simulink model "ab"  (R2023b)
settings: configuration reference "VTOLConfiguration" (kept outside this file)
undefined symbols (not defined in the file): airspeed, CityMission, control, controlParams, ControlSampleTime, CriticalTiltAngle, ddx, ddy, ddz, DiscIntNeverNeededParam, dx, dy, dz, Earth, env, F, FixedWingMission, flightState, fractalcoef, FSState, FWControlParams, HoverMission, iniRoll, initPitch, iniYaw, Light, MIL, p, pitch, q, r, R_LOOKAHEAD, ReferenceFilterDen, ReferenceFilterNum, roll, SensorAAFiltDen, SensorAAFiltNum, tiltIni, TiltScheduleRate, TransitionMission, uavParam, UAVSampleTime, vIni, Vt, WGS84, windVel, X, xGround, Y, yaw, yGround, Z, zGround
libraries: slpidlib x37, simulink x10, uavalgslib x6, mbdriLib x4, robotcorelib x3, aerolibasang x2, aerolibwind2 x2, sharedtransform x2, simulink_extras x2, shared6dof x1, aerolibatmos2 x1, sensorgpslib x1
(part 1 of 7)
settings Model: DataDictionary=VTOLDynamicsData.sldd  Creator=The MathWorks, Inc.  LastModifiedBy=USER
settings ConfigSetRef: SourceName=VTOLConfiguration

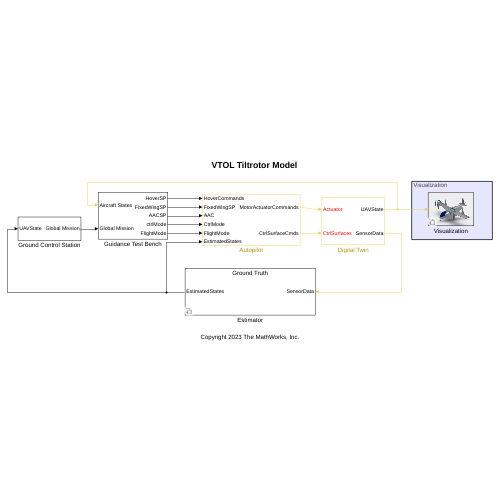
[thumbnail: Simulink's stored preview of the top-level diagram]
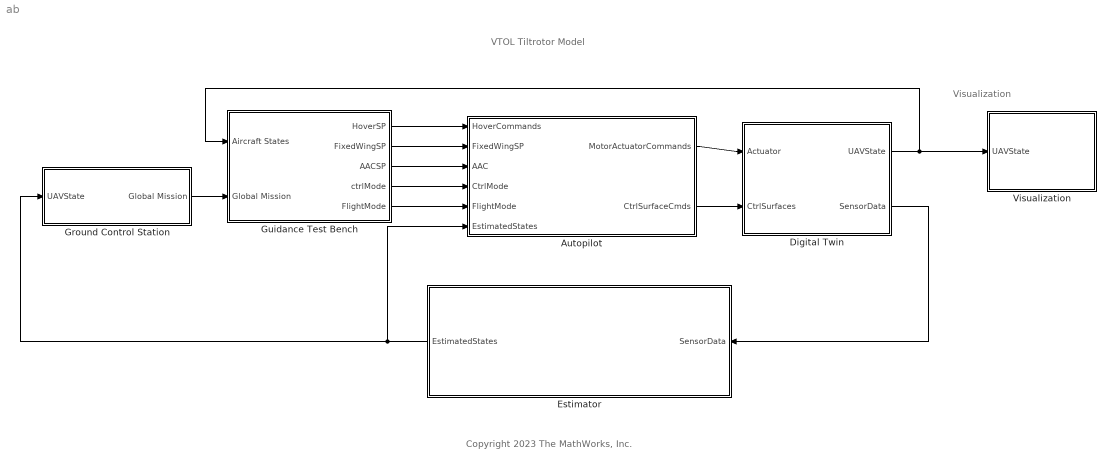
== system ab ==
  note: VTOL Tiltrotor Model
  note: Visualization
  note: Copyright 2023 The MathWorks, Inc.
  Autopilot : Subsystem
  Digital Twin : Subsystem
  Estimator : Subsystem  Variant=on
  Ground Control Station : Subsystem
  Guidance Test Bench : Subsystem
  Visualization : Subsystem  Variant=on  VariantControl=Visualization
      mask Display: image('TiltrotorVisualization.PNG'); % Use "Edit Image" on toolstrip to change.
  wires:
  Autopilot/1(MotorActuatorCommands) -> Digital Twin/1(Actuator)
  Autopilot/2(CtrlSurfaceCmds) -> Digital Twin/2(CtrlSurfaces)
  Digital Twin/2(SensorData) -> Estimator/1(SensorData)
  Guidance Test Bench/1(HoverSP) -> Autopilot/1(HoverCommands)
  Ground Control Station/1(Global Mission) -> Guidance Test Bench/2(Global Mission)
  Guidance Test Bench/2(FixedWingSP) -> Autopilot/2(FixedWingSP)
  Guidance Test Bench/3(AACSP) -> Autopilot/3(AAC)
  Guidance Test Bench/4(ctrlMode) -> Autopilot/4(CtrlMode)
  Guidance Test Bench/5(FlightMode) -> Autopilot/5(FlightMode)
  Digital Twin/1(UAVState) -> Guidance Test Bench/1(Aircraft States), Visualization/1(UAVState)
  Estimator/1(EstimatedStates) -> Autopilot/6(EstimatedStates), Ground Control Station/1(UAVState)

== system ab/Autopilot ==
  HoverCommands : Inport
  FixedWingSP : Inport  Port=2
  AAC : Inport  Port=3
  CtrlMode : Inport  Port=4
  FlightMode : Inport  Port=5
  EstimatedStates : Inport  Port=6
  Bus Selector : BusSelector  OutputSignals=inTransition
  Bus Selector1 : BusSelector  OutputSignals=TransitionCondition
  Bus Selector2 : BusSelector  OutputSignals=w1,w2,w3,w4
  Filter or Estimator : Subsystem
  Fixed Wing Controller : Subsystem  Variant=on  VariantControl=Fixed Wing Controller
  Manual Control : Subsystem
  Multicopter Controller : Subsystem
  Scheduler : Subsystem  SystemSampleTime=0.005
  Scope : Scope  NumInputPorts=4
  Scope1 : Scope
  Tilt Scheduler : Subsystem
  MotorActuatorCommands : Outport
  CtrlSurfaceCmds : Outport  Port=2
  wires:
  EstimatedStates/1 -> Filter or Estimator/1(SensorData)
  Multicopter Controller/1(MixerCommands) -> Scheduler/1(MotorCommands)
  Tilt Scheduler/1(TiltAngle) -> Scheduler/2(TiltSchedule)
  Fixed Wing Controller/1(Actuator) -> Scheduler/6(FixedWingActuators)
  CtrlMode/1 -> Bus Selector1/1, Fixed Wing Controller/2(Control Mode), Bus Selector/1
  Manual Control/1(AERT) -> Fixed Wing Controller/5(AERT)
  Scheduler/1(MotorActuatorCommands) -> Bus Selector2/1, MotorActuatorCommands/1
  Scheduler/2(CtrlSurfaceCommands) -> CtrlSurfaceCmds/1
  HoverCommands/1 -> Multicopter Controller/1(Hover Commands)
  FlightMode/1 -> Scope1/1, Tilt Scheduler/1(FlightMode)
  Filter or Estimator/1(States) -> Multicopter Controller/3(States), Fixed Wing Controller/1(States), Tilt Scheduler/2(States), Scheduler/4(States)
  AAC/1 -> Fixed Wing Controller/3(AAC SP)
  FixedWingSP/1 -> Fixed Wing Controller/4(FixedWingSP)
  [TransitionDone] -> Scheduler/5(TransitionDone)
  Tilt Scheduler/2(FlightState) -> Scheduler/3(FlightState)
  Bus Selector/1 -> Multicopter Controller/2(InTransition)  "<inTransition>"
  Bus Selector1/1 -> [TransitionDone]  "<TransitionCondition>"
  Bus Selector2/1 -> Scope/1  "<w1>"
  Bus Selector2/2 -> Scope/2  "<w2>"
  Bus Selector2/3 -> Scope/3  "<w3>"
  Bus Selector2/4 -> Scope/4  "<w4>"

== system ab/Digital Twin ==
  Actuator : Inport
  CtrlSurfaces : Inport  Port=2
  6DOF (Euler Angles)1 : shared6dof/6DOF (Euler Angles)  units=Metric (MKS)  mtype=Fixed  rep=Euler Angles  xme_0=[xGround, yGround, zGround]  Vm_0=[vIni 0 0]  eul_0=[iniRoll initPitch iniYaw]  pm_0=[0 0 0]  mass_0=6.031  mass_e=0.5  mass_f=2.0  inertia=[uavParam.geom.Ixx 0 0; 0 uavParam.geom.Iyy 0; 0 0 uavParam.geom.Izz]  inertia_e=eye(3)  inertia_f=2*eye(3)  k_quat=1.0  vre_flag=on  abi_flag=on  aMode=0  xme_statename=''  Vm_statename=''  eul_statename=''  quat_statename=''  pm_statename=''  mass_statename=''
  Bus Selector : BusSelector  OutputSignals=RotorParameters.w1,RotorParameters.w2,RotorParameters.w3,RotorParameters.w4
  Force and Moments : Subsystem
  Ground Truth Bus : Subsystem
  Scope : Scope  NumInputPorts=4
  Terminator : Terminator
  Variant Subsystem : Subsystem  Variant=on  VariantControl=Choice
  UAVState : Outport
  SensorData : Outport  Port=2
  wires:
  Force and Moments/1(F) -> 6DOF (Euler Angles)1/1
  Force and Moments/2(M) -> 6DOF (Euler Angles)1/2
  Actuator/1 -> Force and Moments/1(Actuator)
  CtrlSurfaces/1 -> Force and Moments/2(CtrlSurfaces)
  6DOF (Euler Angles)1/1 -> Ground Truth Bus/1(Ve)  "Ve"
  6DOF (Euler Angles)1/2 -> Ground Truth Bus/2(Xe)  "Xe"
  6DOF (Euler Angles)1/3 -> Ground Truth Bus/3(Euler)  "Euler"
  6DOF (Euler Angles)1/4 -> Ground Truth Bus/4(DCMbe)  "DCMbe"
  6DOF (Euler Angles)1/5 -> Ground Truth Bus/5(Vb)  "Vb"
  6DOF (Euler Angles)1/6 -> Ground Truth Bus/6(pqr)  "pqr"
  6DOF (Euler Angles)1/7 -> Terminator/1
  6DOF (Euler Angles)1/8 -> Ground Truth Bus/7(Abb)  "Abb"
  Force and Moments/3(RotorParams) -> Ground Truth Bus/9(RotorParams)  "RotorParams"
  Force and Moments/4(AirData) -> Ground Truth Bus/10(AirData)
  Variant Subsystem/1(SensorData) -> SensorData/1
  6DOF (Euler Angles)1/9 -> Ground Truth Bus/8(Abe)
  Ground Truth Bus/1(Ground Truth) -> Bus Selector/1, UAVState/1, Force and Moments/3(States), Variant Subsystem/1(UAVStates)  "Ground Truth"
  Bus Selector/1 -> Scope/1  "<w1>"
  Bus Selector/2 -> Scope/2  "<w2>"
  Bus Selector/3 -> Scope/3  "<w3>"
  Bus Selector/4 -> Scope/4  "<w4>"

== system ab/Estimator ==
  SensorData : Inport
  Estimation Filter : Subsystem  VariantControl=SensorType==1
  Ground Truth : Subsystem  VariantControl=SensorType==0
  EstimatedStates : Outport

== system ab/Ground Control Station ==
  UAVState : Inport
  Get Flight Mission : Subsystem  Variant=on  VariantControlMode=label  LabelModeActiveChoice=useQGC==0
  Global Mission : Outport
  wires:
  Get Flight Mission/1("Mission ") -> Global Mission/1
  UAVState/1 -> Get Flight Mission/1(UAVState)

== system ab/Guidance Test Bench ==
  Aircraft States : Inport
  Global Mission : Inport  Port=2
  ControlType : Subsystem  Variant=on  VariantControl=Choice
  Rate Transition : RateTransition  OutPortSampleTime=0.005
  "Reference Tracking " : Subsystem
      settings: PortSchema="{\"entries\":[{\"content\":{\"sides\":[{\"content\":{\"connectorIds\":[\"In1\"]},\"type\":\"ConnectorPlacement.EquallySpacedRectSide\",\"uuid\":\"259d5f1e-a362-4dc0-8429-ef92dd781b31\"},{\"content\":{\"connectorIds\":[\"In2\",\"In3\"],\"side\":\"RIGHT\"},\"type\":\"ConnectorPlacement.EquallySpacedRectSide\",\"uuid\":\"8f699bfb-ab92-4bfa-94de-3c6c350a8a94\"},{\"content\":{\"connectorIds\":[],\"side\":\"TOP\"},\"type\":\"ConnectorPlacement.EquallySpacedRectSide\",\"uuid\":\"95dbffc6-e5b7-446a-adcb-afa0cff8c552\"}]},\"type\":\"ConnectorPlacement.EquallySpacedConnector\",\"uuid\":\"e657b5d9-4fa5-41f8-85e3-18a1074ff1cd\"}],\"packageUris\":[\"http://schema.mathworks.com/mf0/Connector/R2020b\"],\"version\":\"1.0\"}"
  HoverSP : Outport
  FixedWingSP : Outport  Port=2
  AACSP : Outport  Port=3
  ctrlMode : Outport  Port=4
  FlightMode : Outport  Port=5
  wires:
  Aircraft States/1 -> Rate Transition/1
  ControlType/1(HoverCmds) -> "Reference Tracking "/2(Position Command), HoverSP/1
  Global Mission/1 -> ControlType/2(Global Mission)
  ControlType/2(FixedWingSP) -> FixedWingSP/1
  ControlType/5(FlightMode) -> FlightMode/1
  ControlType/4(ctrlMode) -> ctrlMode/1
  ControlType/3(AACSP) -> "Reference Tracking "/3(AAC Commands), AACSP/1
  Rate Transition/1 -> "Reference Tracking "/1(State), ControlType/1(Aircraft States)

== system ab/Visualization ==
  UAVState : Inport
  No Visualization : Subsystem  VariantControl=Visualization==0
  Photorealistic : Subsystem  VariantControl=Visualization==2
  Visualization : Subsystem  VariantControl=Visualization==1

== system ab/Autopilot/Filter or Estimator ==
  SensorData : Inport
  States : Outport
  wires:
  SensorData/1 -> States/1

== system ab/Autopilot/Fixed Wing Controller ==
  States : Inport
  Control Mode : Inport  Port=2
  AAC SP : Inport  Port=3
  FixedWingSP : Inport  Port=4
  AERT : Inport  Port=5
  Fixed Wing Controller Simulation : Subsystem  VariantControl=TuningMode == 0
  Fixed Wing Controller Tuning : Subsystem  VariantControl=TuningMode ~= 0
  Actuator : Outport

== system ab/Autopilot/Manual Control ==
  Bus Creator : BusCreator  Inputs=4
  Constant{,1..3} (4 alike) : Constant  Value=0
  AERT : Outport
  wires:
  Constant/1 -> Bus Creator/1  "aileron"
  Constant1/1 -> Bus Creator/2  "throttle"
  Constant2/1 -> Bus Creator/3  "elevator"
  Constant3/1 -> Bus Creator/4  "rudder"
  Bus Creator/1 -> AERT/1

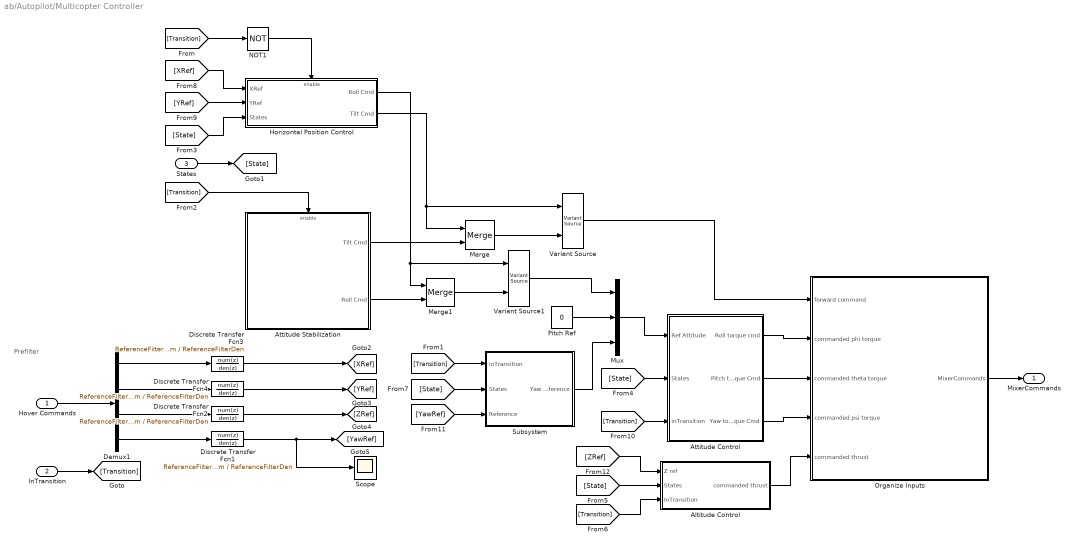
== system ab/Autopilot/Multicopter Controller ==
  note: Prefilter
  Hover Commands : Inport
  InTransition : Inport  Port=2
  States : Inport  Port=3
  Altitude Control : Subsystem
  Attitude Control : Subsystem  Variant=on  VariantControlMode=label  VariantControl=Choice  LabelModeActiveChoice=AttitudeControl==1
  Attitude Stabilization : Subsystem  TreatAsAtomicUnit=on
  Demux1 : Demux
  Discrete Transfer Fcn{1..4} (4 alike) : DiscreteTransferFcn  Numerator=ReferenceFilterNum  Denominator=ReferenceFilterDen
  Horizontal Position Control : Subsystem  TreatAsAtomicUnit=on
  Merge : Merge
  Merge1 : Merge
  Mux : Mux  Inputs=3
  NOT1 : Logic  Operator=NOT  IconShape=distinctive  AllPortsSameDT=off  OutDataTypeStr=boolean
  Organize Inputs : Subsystem
  Pitch Ref : Constant  Value=0
  Scope : Scope
  Subsystem : Subsystem
  Variant Source : VariantSource
  Variant Source1 : VariantSource
  MixerCommands : Outport
  wires:
  [Transition] -> NOT1/1
  [State] -> Horizontal Position Control/3(States)
  Variant Source1/1 -> Mux/1
  States/1 -> [State]
  Hover Commands/1 -> Demux1/1
  InTransition/1 -> [Transition]
  NOT1/1 -> Horizontal Position Control/Enable
  [YRef] -> Horizontal Position Control/2(YRef)
  [XRef] -> Horizontal Position Control/1(XRef)
  Attitude Control/1(Roll torque cmd) -> Organize Inputs/2(commanded phi torque)
  [Transition] -> Attitude Stabilization/Enable
  Demux1/3 -> Discrete Transfer Fcn2/1
  Demux1/1 -> Discrete Transfer Fcn3/1
  [State] -> Altitude Control/2(States)
  Demux1/2 -> Discrete Transfer Fcn4/1
  Discrete Transfer Fcn3/1 -> [XRef]
  Demux1/4 -> Discrete Transfer Fcn1/1
  Horizontal Position Control/1(Roll Cmd) -> Variant Source1/1, Merge1/1
  Horizontal Position Control/2(Tilt Cmd) -> Merge/1, Variant Source/1
  Attitude Control/3(Yaw torque Cmd) -> Organize Inputs/4(commanded psi torque)
  Attitude Stabilization/1(Tilt Cmd) -> Merge/2
  Attitude Control/2(Pitch torque Cmd) -> Organize Inputs/3(commanded theta torque)
  Attitude Stabilization/2(Roll Cmd) -> Merge1/2
  Discrete Transfer Fcn4/1 -> [YRef]
  Merge/1 -> Variant Source/2
  Merge1/1 -> Variant Source1/2
  [Transition] -> Subsystem/1(inTransition)
  [State] -> Subsystem/2(States)
  [YawRef] -> Subsystem/3(Reference)
  Variant Source/1 -> Organize Inputs/1(forward command)
  Pitch Ref/1 -> Mux/2
  Subsystem/1(Yaw Reference) -> Mux/3
  Mux/1 -> Attitude Control/1(Ref Attitude)
  [State] -> Attitude Control/2(States)
  [Transition] -> Attitude Control/3(inTransition)
  [ZRef] -> Altitude Control/1(Z ref)
  [Transition] -> Altitude Control/3(InTransition)
  Altitude Control/1(commanded thrust) -> Organize Inputs/5(commanded thrust)
  Organize Inputs/1(MixerCommands) -> MixerCommands/1
  Discrete Transfer Fcn1/1 -> Scope/1, [YawRef]
  Discrete Transfer Fcn2/1 -> [ZRef]

== system ab/Autopilot/Scheduler ==
  MotorCommands : Inport
  TiltSchedule : Inport  Port=2
  FlightState : Inport  Port=3  OutDataTypeStr=Enum: flightState
  States : Inport  Port=4
  TransitionDone : Inport  Port=5
  FixedWingActuators : Inport  Port=6
  Subsystem : Subsystem  ReferencedSubsystem=FixedWingScheduler
  Subsystem1 : Subsystem  ReferencedSubsystem=MulticopterScheduler
  MotorActuatorCommands : Outport
  CtrlSurfaceCommands : Outport  Port=2  VectorParamsAs1DForOutWhenUnconnected=off
  wires:
  Subsystem/1 -> Subsystem1/2, CtrlSurfaceCommands/1
  FlightState/1 -> Subsystem/1, Subsystem1/1  "Flight State"
  TiltSchedule/1 -> Subsystem1/4
  Subsystem1/1 -> MotorActuatorCommands/1
  MotorCommands/1 -> Subsystem1/3
  FixedWingActuators/1 -> Subsystem/2
  TransitionDone/1 -> Subsystem/3, Subsystem1/5  "Transition Done"
  States/1 -> Subsystem1/6

== system ab/Autopilot/Tilt Scheduler ==
  note: Forward Transition Tilt Mode Manager
  note: Back Transition Tilt Mode Manager
  FlightMode : Inport
  States : Inport  Port=2
  Back Transition Scheduler : Subsystem
  Forward Transition Scheduler : Subsystem
  TiltAngle : Outport
  FlightState : Outport  Port=2
  wires:
  States/1 -> Back Transition Scheduler/3(States)
  Back Transition Scheduler/1(TiltAngle) -> TiltAngle/1
  FlightMode/1 -> Back Transition Scheduler/2(FlightMode), Forward Transition Scheduler/1(FlightMode)
  Forward Transition Scheduler/1(FlightState) -> FlightState/1
  Forward Transition Scheduler/2(Tilt Schedule) -> Back Transition Scheduler/1(Tilt Schedule)

== system ab/Digital Twin/Force and Moments ==
  Actuator : Inport
  CtrlSurfaces : Inport  Port=2
  States : Inport  Port=3
  Add : Sum  Inputs=++++
  Add1 : Sum
  AeroSwitch : Constant
  Aerodynamic Drag : Subsystem
  Aerodynamic Forces : Subsystem
  Bus Selector : BusSelector  OutputSignals=DCMbe,Vb
  Bus Selector3 : BusSelector  OutputSignals=Xe,Euler
  Constant4 : Constant  Value=0
  Constant5 : Constant  Value=0
  Gravity : Subsystem
  Propulsion : Subsystem
  Switch : Switch  Criteria=u2 > Threshold  SaturateOnIntegerOverflow=off  InputSameDT=off
  Switch1 : Switch  Criteria=u2 > Threshold  SaturateOnIntegerOverflow=off  InputSameDT=off
  Weather Model : Subsystem  Variant=on  VariantControl=Weather Model
  F : Outport
  M : Outport  Port=2
  RotorParams : Outport  Port=3
  AirData : Outport  Port=4
  wires:
  Bus Selector/1 -> Gravity/1(DCM_be), Aerodynamic Drag/1(DCM_be)  "<DCMbe>"
  Propulsion/3(F) -> Add/1
  Gravity/1(F_g) -> Add/2  "Gravity Force"
  Aerodynamic Drag/1(F_d) -> Add/4  "Drag Force"
  Bus Selector/2 -> Aerodynamic Drag/2(Vb)  "<Vb>"
  Add/1 -> F/1
  States/1 -> Bus Selector3/1, Bus Selector/1, Aerodynamic Forces/4(UAVState), Propulsion/2(States)  "States"
  CtrlSurfaces/1 -> Aerodynamic Forces/3(CtrlSurfaces)
  Add1/1 -> M/1
  Propulsion/2(M) -> Add1/2
  [AeroForce] -> Add/3  "Aerodynamic Force"
  Aerodynamic Forces/2(F) -> Switch/1
  Switch/1 -> [AeroForce]
  Constant4/1 -> Switch/3
  AeroSwitch/1 -> Switch/2, Switch1/2
  Constant5/1 -> Switch1/3
  Switch1/1 -> Add1/1, [AeroMoment]
  Aerodynamic Forces/3(M) -> Switch1/1
  Actuator/1 -> Propulsion/1(Actuator)
  Propulsion/1(RotorParameters) -> RotorParams/1
  Aerodynamic Forces/1(AirData) -> AirData/1, Weather Model/1(AirData)  "Air Data"
  Bus Selector3/1 -> Weather Model/2(Xe)  "<Xe>"
  Bus Selector3/2 -> Weather Model/3(Euler)  "<Euler>"
  Weather Model/1(Wind_e) -> Aerodynamic Forces/1(Wind_e)
  Weather Model/2(Rho) -> Aerodynamic Forces/2(Rho)

== system ab/Digital Twin/Ground Truth Bus ==
  Ve : Inport
  Xe : Inport  Port=2
  Euler : Inport  Port=3
  DCMbe : Inport  Port=4
  Vb : Inport  Port=5
  pqr : Inport  Port=6
  Abb : Inport  Port=7
  Abe : Inport  Port=8
  RotorParams : Inport  Port=9
  AirData : Inport  Port=10
  Bus Creator : BusCreator  Inputs=13
  Bus Selector : BusSelector  OutputSignals=airspeed
  Direction Cosine Matrix to Quaternions : sharedtransform/Direction Cosine Matrix  to Quaternions  aMode=0  action=None  tolerance=eps(2)
      settings: LibrarySourceBlock=|
      | aerolibtransform2/Direction Cosine Matrix
      | to Quaternions
  MATLAB Function1 : MATLAB Function  TreatAsAtomicUnit=on
  Ground Truth : Outport
  wires:
  pqr/1 -> Bus Creator/6
  Xe/1 -> Bus Creator/2
  Bus Creator/1 -> Ground Truth/1
  DCMbe/1 -> Direction Cosine Matrix to Quaternions/1, Bus Creator/4
  Euler/1 -> Bus Creator/3
  Vb/1 -> Bus Creator/5
  Abb/1 -> Bus Creator/7
  AirData/1 -> Bus Selector/1
  Bus Selector/1 -> Bus Creator/9  "<airspeed>"
  Direction Cosine Matrix to Quaternions/1 -> Bus Creator/10  "q"
  RotorParams/1 -> Bus Creator/8  "RotorParameters"
  Abe/1 -> Bus Creator/11  "Abe"
  MATLAB Function1/2(gndSpeed) -> Bus Creator/13  "gndspeed"
  MATLAB Function1/1(course) -> Bus Creator/12  "course"
  Ve/1 -> MATLAB Function1/1(vxyz), Bus Creator/1

== system ab/Digital Twin/Variant Subsystem ==
  UAVStates : Inport
  No Sensors : Subsystem  VariantControl=SensorType==0
  Sensors : Subsystem  VariantControl=SensorType==1
  SensorData : Outport

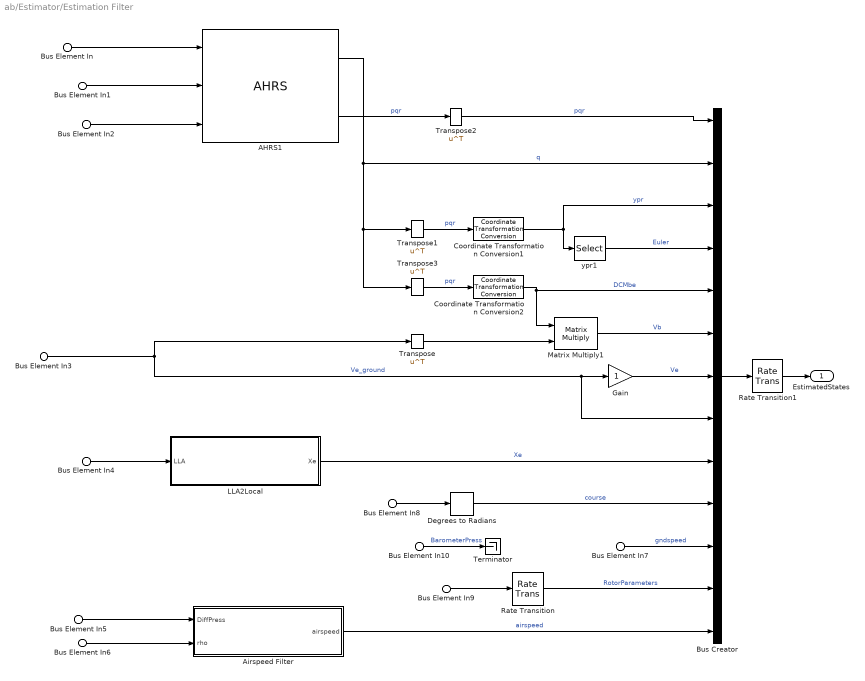
== system ab/Estimator/Estimation Filter ==
  Bus Element In : Inport  PortName=SensorData  Element=Abb
  Bus Element In1 : Inport  PortName=SensorData  Element=Gyro
  Bus Element In2 : Inport  PortName=SensorData  Element=Mag
  Bus Element In3 : Inport  PortName=SensorData  Element=GPSVelocity
  Bus Element In4 : Inport  PortName=SensorData  Element=LLA
  Bus Element In6 : Inport  PortName=SensorData  Element=rho
  Bus Element In5 : Inport  PortName=SensorData  Element=DiffPress
  Bus Element In7 : Inport  PortName=SensorData  Element=GPSGroundSpeed
  Bus Element In8 : Inport  PortName=SensorData  Element=GPSCourse
  Bus Element In9 : Inport  PortName=SensorData  Element=RotorParameters
  Bus Element In10 : Inport  PortName=SensorData  Element=BarometerPress
  AHRS1 : mspfiltlib/AHRS  DispRefFrame=NED  DecimationFactor=1  InitialProcessNoise=ahrsfilter.defaultProcessNoise  OrientationFormat=quaternion  SimulateUsing=Code generation  AccelerometerNoise=0.0001924722  GyroscopeNoise=9.1385e-5  MagnetometerNoise=0.1  GyroscopeDriftNoise=3.0462e-13  LinearAccelerationNoise=0.0096236100000000012  MagneticDisturbanceNoise=0.5  LinearAccelerationDecayFactor=0.998  MagneticDisturbanceDecayFactor=0.5  ExpectedMagneticFieldStrength=40
  Airspeed Filter : Subsystem
  Bus Creator : BusCreator  Inputs=13
  Coordinate Transformation Conversion1 : robotcorelib/Coordinate Transformation Conversion  InputRepresentation=Quaternion  InputEulerSequence=ZYX  ShowTrVecInputPort=on  OutputRepresentation=Euler Angles  OutputEulerSequence=ZYX  ShowTrVecOutputPort=on  SimulateUsing=Interpreted execution
      settings: LibrarySourceBlock=navlib/Utilities/Coordinate Transformation Conversion
  Coordinate Transformation Conversion2 : robotcorelib/Coordinate Transformation Conversion  InputRepresentation=Quaternion  InputEulerSequence=ZYX  ShowTrVecInputPort=on  OutputRepresentation=Rotation Matrix  OutputEulerSequence=ZYX  ShowTrVecOutputPort=on  SimulateUsing=Interpreted execution
      settings: LibrarySourceBlock=navlib/Utilities/Coordinate Transformation Conversion
  Degrees to Radians : simulink_extras/Transformations/Degrees to Radians
  Gain : Gain
  LLA2Local : Subsystem
  Matrix Multiply1 : Product  Multiplication=Matrix(*)
  Rate Transition : RateTransition  OutPortSampleTime=0.001
  Rate Transition1 : RateTransition
  Terminator : Terminator
  Transpose{,1..3} (4 alike) : Math  Operator=transpose
  ypr1 : Selector  InputPortWidth=3  IndexOptions=Index vector (dialog)  Indices=[3 2 1]  OutputSizes=1
  EstimatedStates : Outport
  wires:
  AHRS1/2 -> Transpose2/1  "pqr"
  Bus Element In/1 -> AHRS1/1
  Bus Element In1/1 -> AHRS1/2
  Bus Element In2/1 -> AHRS1/3
  Transpose2/1 -> Bus Creator/1  "pqr"
  AHRS1/1 -> Transpose3/1, Transpose1/1, Bus Creator/2  "q"
  Transpose1/1 -> Coordinate Transformation Conversion1/1  "pqr"
  Coordinate Transformation Conversion1/1 -> Bus Creator/3, ypr1/1  "ypr"
  Bus Element In3/1 -> Transpose/1, Bus Creator/8, Gain/1  "Ve_ground"
  Coordinate Transformation Conversion2/1 -> Bus Creator/5, Matrix Multiply1/1  "DCMbe"
  Bus Element In4/1 -> LLA2Local/1(LLA)
  LLA2Local/1(Xe) -> Bus Creator/9  "Xe"
  Matrix Multiply1/1 -> Bus Creator/6  "Vb"
  Bus Element In8/1 -> Degrees to Radians/1
  Bus Element In7/1 -> Bus Creator/11  "gndspeed"
  Bus Element In10/1 -> Terminator/1  "BarometerPress"
  Bus Element In5/1 -> Airspeed Filter/1(DiffPress)
  Bus Element In9/1 -> Rate Transition/1
  Bus Element In6/1 -> Airspeed Filter/2(rho)
  Airspeed Filter/1(airspeed) -> Bus Creator/13  "airspeed"
  ypr1/1 -> Bus Creator/4  "Euler"
  Transpose3/1 -> Coordinate Transformation Conversion2/1  "pqr"
  Degrees to Radians/1 -> Bus Creator/10  "course"
  Rate Transition/1 -> Bus Creator/12  "RotorParameters"
  Transpose/1 -> Matrix Multiply1/2
  Bus Creator/1 -> Rate Transition1/1
  Rate Transition1/1 -> EstimatedStates/1
  Gain/1 -> Bus Creator/7  "Ve"

== system ab/Estimator/Ground Truth ==
  SensorData : Inport
  Rate Transition : RateTransition  OutPortSampleTime=0.005
  EstimatedStates : Outport
  wires:
  SensorData/1 -> Rate Transition/1
  Rate Transition/1 -> EstimatedStates/1

== system ab/Ground Control Station/Get Flight Mission ==
  UAVState : Inport
  noQGC : Subsystem  TreatAsAtomicUnit=on  SystemSampleTime=UAVSampleTime*4  VariantControl=useQGC==0
  "Mission " : Outport

== system ab/Guidance Test Bench/ControlType ==
  Aircraft States : Inport
  Global Mission : Inport  Port=2
  Guidance Testbench : Subsystem  TreatAsAtomicUnit=on  VariantControl=TestMode==1
  Manual Control : Subsystem  TreatAsAtomicUnit=on  VariantControl=TestMode==0
  HoverCmds : Outport
  FixedWingSP : Outport  Port=2
  AACSP : Outport  Port=3
  ctrlMode : Outport  Port=4
  FlightMode : Outport  Port=5

== system ab/Guidance Test Bench/Reference Tracking  ==
  State : Inport
  Position Command : Inport  Port=2
  AAC Commands : Inport  Port=3
  Fixed Wing Reference : Subsystem
  Hover Reference : Subsystem
  Transition Reference : Subsystem
  wires:
  State/1 -> Transition Reference/1(States), Fixed Wing Reference/2(States), Hover Reference/2(Position Reference)
  AAC Commands/1 -> Fixed Wing Reference/1(AAC Commands)
  Position Command/1 -> Hover Reference/1(Position Command)

== system ab/Visualization/No Visualization ==
  UAVState : Inport
  Terminator : Terminator
  wires:
  UAVState/1 -> Terminator/1

== system ab/Visualization/Photorealistic ==
  UAVState : Inport
  Bus Creator : BusCreator  Inputs=6
  Bus Selector : BusSelector  OutputSignals=Euler,Xe
  Demux : Demux  Outputs=3
  Demux1 : Demux  Outputs=3
  Prepare UAV Data : Subsystem
  Simulation 3D Scene Configuration : sim3dlib/Simulation 3D Scene Configuration  Priority=0  ProjectFormat=Unreal Editor  SceneDesc=US city block  ProjectName=I:\29\vdubey.MergedFixedWingReview\matlab\toolbox\shared\sim3d_projects\automotive_project_windows\UE\WindowsNoEditor\VehicleSimulation.exe  ScenePath=/Game/Maps/USCityBlock  UEProjPath=C:\Documents\project\AutoVrtlEnv\AutoVrtlEnv.uproject  EnableOpenDRIVE=off  vehTagList={'Scene Origin';'VTOL_Vehicle'}  vehTag=VTOL_Vehicle  FreeCameraInitialTranslation=[0, 0, 0]  FreeCameraDefaultInitialTranslation=[-6, 0, 2]  FreeCameraInitialRotation=[0, 0, 0]  FreeCameraDefaultInitialRotation=[0, -15, 0]  OpVisEn=off  Ts=1/10  EnableWindow=on  EnableRemoteAccess=off  EnableWeather=off  SunAltitude=40.0  SunAzimuth=90  clouds=10  wind=1  fog=0  rain=0  EnableGeospatial=off  OriginHeight=200  OriginLatitude=40.744652  OriginLongitude=-73.988864  MapStyle=Aerial  AdditionalAssetIDs=[]  UseAdvancedSunSky=off  SolarTime=11  TimeZone=-5  Day=21  Month=9  Year=2022  UseDaylightSavingTime=on  DSTStartDay=10  DSTStartMonth=3  DSTEndDay=3  DSTEndMonth=11  DSTSwitchHour=2  sensorTag=MainCamera2  sensorId=2  sensorName=MainCamera2  mountLoc=Origin  offsetFlag=off  tmountOffset=[0, 0, 0]  rmountOffset=[0, 0, 0]  HorizontalResolution=1280  VerticalResolution=720  HorizontalFOV=60  mountPoint=[0 0 0]  mountOrientation=[0 0 0]  aMode=4  ID=2  GeoTrigger=Inactive
      settings: LibrarySourceBlock=uavsim3dlib/Simulation 3D Scene Configuration
  Simulation 3D UAV Vehicle : uavsim3dlib/Simulation 3D UAV Vehicle  Priority=-1  Mesh=Custom  MeshPath=SkeletalMesh'/Game/Maps/VTOLDEMO/VTOLAsset.VTOLAsset'  Color=Black  ActorName=VTOL_Vehicle  UseGlobalFrame=off  InitialTranslation=[0 0 0]  InitialRotation=[0 0 0]  InitialTranslationGlobal=[0 0 0]  InitialGeoOrigin=[0 0 0]  InitialRotationGlobal=[0 0 0]  SampleTime=0.1  ActorType=SimulinkVehicle  ID=C  aMode=4  ActorTag=VTOL_Vehicle
  wires:
  UAVState/1 -> Bus Selector/1
  Bus Selector/2 -> Demux1/1  "<Xe>"
  Bus Selector/1 -> Demux/1  "<Euler>"
  Prepare UAV Data/2(Rotation) -> Simulation 3D UAV Vehicle/2
  Demux/1 -> Bus Creator/1  "roll"
  Demux/3 -> Bus Creator/3  "yaw"
  Demux1/1 -> Bus Creator/4  "x"
  Demux1/2 -> Bus Creator/5  "y"
  Bus Creator/1 -> Prepare UAV Data/1(UAVState)
  Demux1/3 -> Bus Creator/6  "z"
  Demux/2 -> Bus Creator/2  "pitch"
  Prepare UAV Data/1(Translation) -> Simulation 3D UAV Vehicle/1

== system ab/Visualization/Visualization ==
  UAVState : Inport
  Bus Selector : BusSelector  OutputSignals=Xe,q,RotorParameters.Rotor A,RotorParameters.Rotor B
  Gain : Gain  Gain=0
  Subsystem : Subsystem
  Trajectory : uavutilslib/UAV Animation  UAVType=FixedWing  UAVSize=5  InertialZDirection=Down  SampleTime=0.1
  wires:
  Bus Selector/2 -> Subsystem/2(<q>), Trajectory/2  "<q>"
  Bus Selector/1 -> Trajectory/1, Gain/1  "<Xe>"
  Gain/1 -> Subsystem/1(<Xe>)
  UAVState/1 -> Bus Selector/1
  Bus Selector/3 -> Subsystem/3(RotorA)  "<Rotor A>"
  Bus Selector/4 -> Subsystem/4(RotorB)  "<Rotor B>"

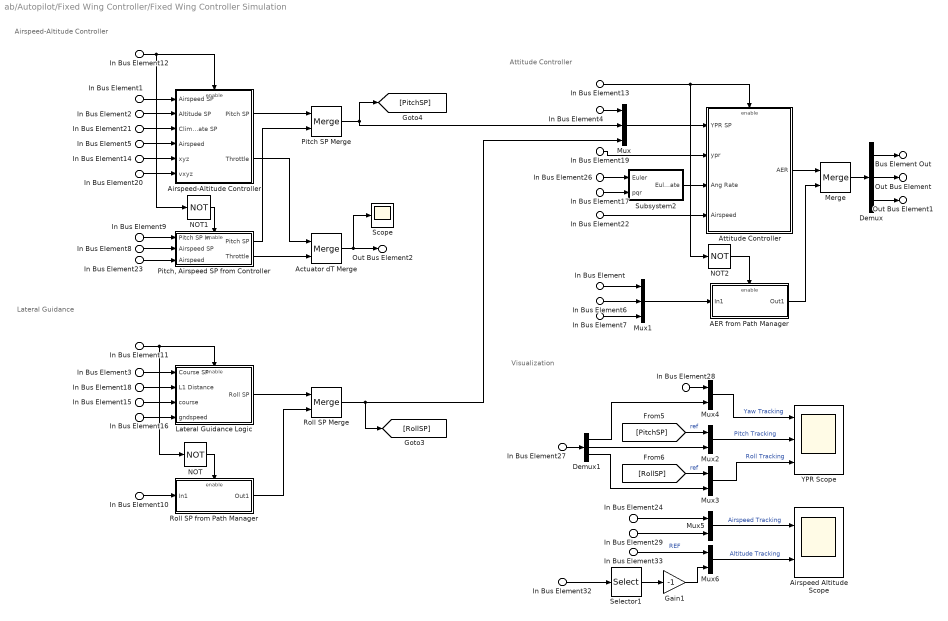
== system ab/Autopilot/Fixed Wing Controller/Fixed Wing Controller Simulation ==
  note: Attitude Controller
  note: Lateral Guidance
  note: Airspeed-Altitude Controller
  note: Visualization
  In Bus Element14 : Inport  PortName=States  Element=Xe
  In Bus Element32 : Inport  PortName=States  Element=Xe
  In Bus Element15 : Inport  PortName=States  Element=course
  In Bus Element17 : Inport  PortName=States  Element=pqr
  In Bus Element{5,22..23,29} (4 alike) : Inport  PortName=States  Element=airspeed
  In Bus Element19 : Inport  PortName=States  Element=ypr
  In Bus Element27 : Inport  PortName=States  Element=ypr
  In Bus Element16 : Inport  PortName=States  Element=gndspeed
  In Bus Element26 : Inport  PortName=States  Element=Euler
  In Bus Element20 : Inport  PortName=States  Element=Ve_ground
  In Bus Element11 : Inport  Port=2  PortName=Control Mode  Element=lateralGuidance
  In Bus Element12 : Inport  Port=2  PortName=Control Mode  Element=airspeedAltitude
  In Bus Element13 : Inport  Port=2  PortName=Control Mode  Element=attitude
  In Bus Element1 : Inport  Port=3  PortName=AAC SP  Element=airspeed
  In Bus Element24 : Inport  Port=3  PortName=AAC SP  Element=airspeed
  In Bus Element2 : Inport  Port=3  PortName=AAC SP  Element=altitude
  In Bus Element33 : Inport  Port=3  PortName=AAC SP  Element=altitude
  In Bus Element18 : Inport  Port=3  PortName=AAC SP  Element=L1
  In Bus Element21 : Inport  Port=3  PortName=AAC SP  Element=course
  In Bus Element3 : Inport  Port=3  PortName=AAC SP  Element=course
  In Bus Element4 : Inport  Port=4  PortName=FixedWingSP  Element=yaw
  In Bus Element28 : Inport  Port=4  PortName=FixedWingSP  Element=yaw
  In Bus Element9 : Inport  Port=4  PortName=FixedWingSP  Element=pitch
  In Bus Element10 : Inport  Port=4  PortName=FixedWingSP  Element=roll
  In Bus Element8 : Inport  Port=4  PortName=FixedWingSP  Element=airspeed
  In Bus Element : Inport  Port=5  PortName=AERT  Element=aileron
  In Bus Element6 : Inport  Port=5  PortName=AERT  Element=elevator
  In Bus Element7 : Inport  Port=5  PortName=AERT  Element=rudder
  AER from Path Manager : Subsystem  TreatAsAtomicUnit=on
  Actuator dT Merge : Merge
  Airspeed Altitude Scope : Scope  NumInputPorts=2
  Airspeed-Altitude Controller : Subsystem
  Attitude Controller : Subsystem
  Demux : Demux  Outputs=3
  Demux1 : Demux  Outputs=3
  Gain1 : Gain  Gain=-1
  Lateral Guidance Logic : Subsystem
  Merge : Merge
  Mux : Mux  Inputs=3
  Mux1 : Mux  Inputs=3
  Mux{2..6} (5 alike) : Mux  Inputs=2
  NOT : Logic  Operator=NOT  IconShape=distinctive  AllPortsSameDT=off  OutDataTypeStr=boolean
  NOT1 : Logic  Operator=NOT  IconShape=distinctive  AllPortsSameDT=off  OutDataTypeStr=boolean
  NOT2 : Logic  Operator=NOT  IconShape=distinctive  AllPortsSameDT=off  OutDataTypeStr=boolean
  Pitch SP Merge : Merge
  "Pitch, Airspeed SP from Controller" : Subsystem  TreatAsAtomicUnit=on
  Roll SP Merge : Merge
  Roll SP from Path Manager : Subsystem  TreatAsAtomicUnit=on
  Scope : Scope
  Selector1 : Selector  InputPortWidth=3  IndexOptions=Index vector (dialog)  Indices=[3]  OutputSizes=1
  Subsystem2 : Subsystem
  YPR Scope : Scope  NumInputPorts=3
  Bus Element Out : Outport  PortName=Actuator  Element=dA
  Out Bus Element : Outport  PortName=Actuator  Element=dE
  Out Bus Element1 : Outport  PortName=Actuator  Element=dR
  Out Bus Element2 : Outport  PortName=Actuator  Element=dT
  wires:
  [PitchSP] -> Mux2/1  "ref"
  In Bus Element24/1 -> Mux5/1
  Mux6/1 -> Airspeed Altitude Scope/2  "Altitude Tracking"
  Pitch SP Merge/1 -> Mux/2, [PitchSP]
  Demux/2 -> Out Bus Element/1
  Airspeed-Altitude Controller/1(Pitch SP) -> Pitch SP Merge/1
  In Bus Element18/1 -> Lateral Guidance Logic/2(L1 Distance)
  In Bus Element1/1 -> Airspeed-Altitude Controller/1(Airspeed SP)
  In Bus Element17/1 -> Subsystem2/2(pqr)
  Demux1/3 -> Mux3/2
  Demux1/1 -> Mux4/2
  Actuator dT Merge/1 -> Scope/1, Out Bus Element2/1
  In Bus Element26/1 -> Subsystem2/1(Euler)
  In Bus Element11/1 -> Lateral Guidance Logic/Enable, NOT/1
  Subsystem2/1(Euler Rate) -> Attitude Controller/3(Ang Rate)
  In Bus Element13/1 -> NOT2/1, Attitude Controller/Enable
  In Bus Element3/1 -> Lateral Guidance Logic/1(Course SP)
  In Bus Element22/1 -> Attitude Controller/4(Airspeed)
  Demux/3 -> Out Bus Element1/1
  Roll SP from Path Manager/1(Out1) -> Roll SP Merge/2
  In Bus Element4/1 -> Mux/1
  In Bus Element14/1 -> Airspeed-Altitude Controller/5(xyz)
  In Bus Element15/1 -> Lateral Guidance Logic/3(course)
  In Bus Element27/1 -> Demux1/1
  In Bus Element6/1 -> Mux1/2
  Mux1/1 -> AER from Path Manager/1(In1)
  Airspeed-Altitude Controller/2(Throttle) -> Actuator dT Merge/1
  "Pitch, Airspeed SP from Controller"/1(Pitch SP) -> Pitch SP Merge/2
  In Bus Element16/1 -> Lateral Guidance Logic/4(gndspeed)
  "Pitch, Airspeed SP from Controller"/2(Throttle) -> Actuator dT Merge/2
  In Bus Element/1 -> Mux1/1
  In Bus Element2/1 -> Airspeed-Altitude Controller/2(Altitude SP)
  In Bus Element7/1 -> Mux1/3
  In Bus Element9/1 -> "Pitch, Airspeed SP from Controller"/1(Pitch SP In)
  Merge/1 -> Demux/1
  In Bus Element10/1 -> Roll SP from Path Manager/1(In1)
  Mux/1 -> Attitude Controller/1(YPR SP)
  Attitude Controller/1(AER) -> Merge/1
  Demux1/2 -> Mux2/2
  NOT1/1 -> "Pitch, Airspeed SP from Controller"/Enable
  Gain1/1 -> Mux6/2
  In Bus Element8/1 -> "Pitch, Airspeed SP from Controller"/2(Airspeed SP)
  In Bus Element33/1 -> Mux6/1  "REF"
  In Bus Element20/1 -> Airspeed-Altitude Controller/6(vxyz)
  Mux3/1 -> YPR Scope/3  "Roll Tracking"
  Selector1/1 -> Gain1/1
  In Bus Element19/1 -> Attitude Controller/2(ypr)
  In Bus Element32/1 -> Selector1/1
  NOT2/1 -> AER from Path Manager/Enable
  In Bus Element23/1 -> "Pitch, Airspeed SP from Controller"/3(Airspeed)
  In Bus Element29/1 -> Mux5/2
  Lateral Guidance Logic/1(Roll SP) -> Roll SP Merge/1
  In Bus Element28/1 -> Mux4/1
  NOT/1 -> Roll SP from Path Manager/Enable
  AER from Path Manager/1(Out1) -> Merge/2
  In Bus Element5/1 -> Airspeed-Altitude Controller/4(Airspeed)
  Demux/1 -> Bus Element Out/1
  In Bus Element21/1 -> Airspeed-Altitude Controller/3(Climb Rate SP)
  Mux5/1 -> Airspeed Altitude Scope/1  "Airspeed Tracking"
  Mux2/1 -> YPR Scope/2  "Pitch Tracking"
  Roll SP Merge/1 -> [RollSP], Mux/3
  In Bus Element12/1 -> Airspeed-Altitude Controller/Enable, NOT1/1
  [RollSP] -> Mux3/1  "ref"
  Mux4/1 -> YPR Scope/1  "Yaw Tracking"

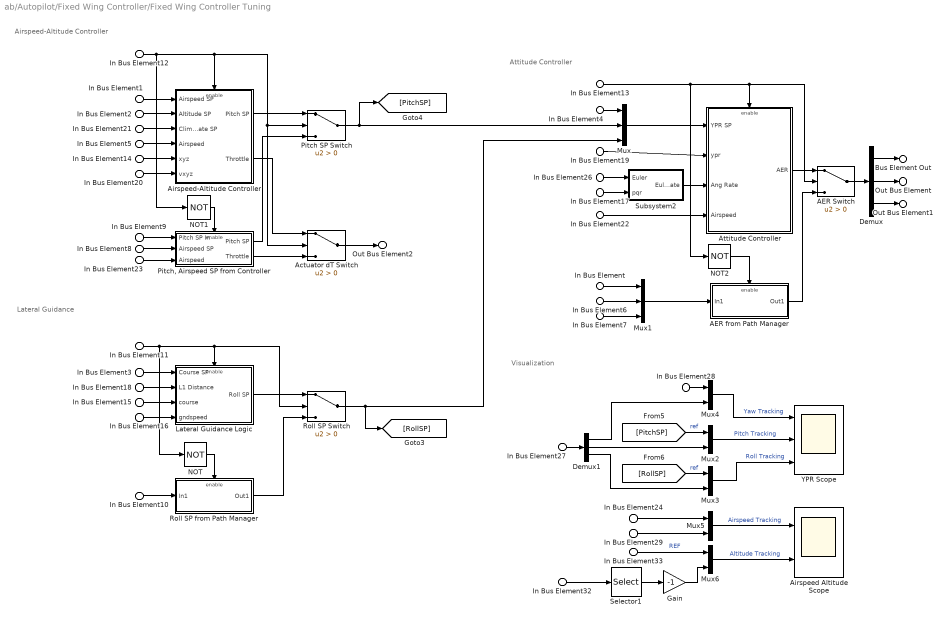
== system ab/Autopilot/Fixed Wing Controller/Fixed Wing Controller Tuning ==
  note: Visualization
  note: Attitude Controller
  note: Airspeed-Altitude Controller
  note: Lateral Guidance
  In Bus Element14 : Inport  PortName=States  Element=Xe
  In Bus Element32 : Inport  PortName=States  Element=Xe
  In Bus Element15 : Inport  PortName=States  Element=course
  In Bus Element17 : Inport  PortName=States  Element=pqr
  In Bus Element{5,22..23,29} (4 alike) : Inport  PortName=States  Element=airspeed
  In Bus Element19 : Inport  PortName=States  Element=ypr
  In Bus Element27 : Inport  PortName=States  Element=ypr
  In Bus Element16 : Inport  PortName=States  Element=gndspeed
  In Bus Element26 : Inport  PortName=States  Element=Euler
  In Bus Element20 : Inport  PortName=States  Element=Ve_ground
  In Bus Element11 : Inport  Port=2  PortName=Control Mode  Element=lateralGuidance
  In Bus Element12 : Inport  Port=2  PortName=Control Mode  Element=airspeedAltitude
  In Bus Element13 : Inport  Port=2  PortName=Control Mode  Element=attitude
  In Bus Element1 : Inport  Port=3  PortName=AAC SP  Element=airspeed
  In Bus Element24 : Inport  Port=3  PortName=AAC SP  Element=airspeed
  In Bus Element2 : Inport  Port=3  PortName=AAC SP  Element=altitude
  In Bus Element33 : Inport  Port=3  PortName=AAC SP  Element=altitude
  In Bus Element18 : Inport  Port=3  PortName=AAC SP  Element=L1
  In Bus Element21 : Inport  Port=3  PortName=AAC SP  Element=course
  In Bus Element3 : Inport  Port=3  PortName=AAC SP  Element=course
  In Bus Element4 : Inport  Port=4  PortName=FixedWingSP  Element=yaw
  In Bus Element28 : Inport  Port=4  PortName=FixedWingSP  Element=yaw
  In Bus Element9 : Inport  Port=4  PortName=FixedWingSP  Element=pitch
  In Bus Element10 : Inport  Port=4  PortName=FixedWingSP  Element=roll
  In Bus Element8 : Inport  Port=4  PortName=FixedWingSP  Element=airspeed
  In Bus Element : Inport  Port=5  PortName=AERT  Element=aileron
  In Bus Element6 : Inport  Port=5  PortName=AERT  Element=elevator
  In Bus Element7 : Inport  Port=5  PortName=AERT  Element=rudder
  AER Switch : Switch  Criteria=u2 > Threshold  SaturateOnIntegerOverflow=off  InputSameDT=off
  AER from Path Manager : Subsystem  TreatAsAtomicUnit=on
  Actuator dT Switch : Switch  Criteria=u2 > Threshold  SaturateOnIntegerOverflow=off  InputSameDT=off
  Airspeed Altitude Scope : Scope  NumInputPorts=2
  Airspeed-Altitude Controller : Subsystem
  Attitude Controller : Subsystem
  Demux : Demux  Outputs=3
  Demux1 : Demux  Outputs=3
  Gain : Gain  Gain=-1
  Lateral Guidance Logic : Subsystem
  Mux : Mux  Inputs=3
  Mux1 : Mux  Inputs=3
  Mux{2..6} (5 alike) : Mux  Inputs=2
  NOT : Logic  Operator=NOT  IconShape=distinctive  AllPortsSameDT=off  OutDataTypeStr=boolean
  NOT1 : Logic  Operator=NOT  IconShape=distinctive  AllPortsSameDT=off  OutDataTypeStr=boolean
  NOT2 : Logic  Operator=NOT  IconShape=distinctive  AllPortsSameDT=off  OutDataTypeStr=boolean
  Pitch SP Switch : Switch  Criteria=u2 > Threshold  SaturateOnIntegerOverflow=off  InputSameDT=off
  "Pitch, Airspeed SP from Controller" : Subsystem  TreatAsAtomicUnit=on
  Roll SP Switch : Switch  Criteria=u2 > Threshold  SaturateOnIntegerOverflow=off  InputSameDT=off
  Roll SP from Path Manager : Subsystem  TreatAsAtomicUnit=on
  Selector1 : Selector  InputPortWidth=3  IndexOptions=Index vector (dialog)  Indices=[3]  OutputSizes=1
  Subsystem2 : Subsystem
  YPR Scope : Scope  NumInputPorts=3
  Bus Element Out : Outport  PortName=Actuator  Element=dA
  Out Bus Element : Outport  PortName=Actuator  Element=dE
  Out Bus Element1 : Outport  PortName=Actuator  Element=dR
  Out Bus Element2 : Outport  PortName=Actuator  Element=dT
  wires:
  Mux/1 -> Attitude Controller/1(YPR SP)
  Attitude Controller/1(AER) -> AER Switch/1
  AER Switch/1 -> Demux/1
  Demux/1 -> Bus Element Out/1
  NOT/1 -> Roll SP from Path Manager/Enable
  Lateral Guidance Logic/1(Roll SP) -> Roll SP Switch/1
  Roll SP from Path Manager/1(Out1) -> Roll SP Switch/3
  NOT1/1 -> "Pitch, Airspeed SP from Controller"/Enable
  In Bus Element8/1 -> "Pitch, Airspeed SP from Controller"/2(Airspeed SP)
  "Pitch, Airspeed SP from Controller"/1(Pitch SP) -> Pitch SP Switch/3
  Airspeed-Altitude Controller/2(Throttle) -> Actuator dT Switch/1
  "Pitch, Airspeed SP from Controller"/2(Throttle) -> Actuator dT Switch/3
  Mux1/1 -> AER from Path Manager/1(In1)
  AER from Path Manager/1(Out1) -> AER Switch/3
  NOT2/1 -> AER from Path Manager/Enable
  In Bus Element/1 -> Mux1/1
  In Bus Element6/1 -> Mux1/2
  In Bus Element7/1 -> Mux1/3
  In Bus Element9/1 -> "Pitch, Airspeed SP from Controller"/1(Pitch SP In)
  In Bus Element10/1 -> Roll SP from Path Manager/1(In1)
  In Bus Element11/1 -> Roll SP Switch/2, Lateral Guidance Logic/Enable, NOT/1
  In Bus Element18/1 -> Lateral Guidance Logic/2(L1 Distance)
  In Bus Element14/1 -> Airspeed-Altitude Controller/5(xyz)
  In Bus Element19/1 -> Attitude Controller/2(ypr)
  In Bus Element16/1 -> Lateral Guidance Logic/4(gndspeed)
  In Bus Element5/1 -> Airspeed-Altitude Controller/4(Airspeed)
  In Bus Element12/1 -> Actuator dT Switch/2, Pitch SP Switch/2, Airspeed-Altitude Controller/Enable, NOT1/1
  In Bus Element2/1 -> Airspeed-Altitude Controller/2(Altitude SP)
  Roll SP Switch/1 -> Mux/3, [RollSP]
  In Bus Element15/1 -> Lateral Guidance Logic/3(course)
  Demux/3 -> Out Bus Element1/1
  In Bus Element13/1 -> NOT2/1, AER Switch/2, Attitude Controller/Enable
  In Bus Element4/1 -> Mux/1
  In Bus Element22/1 -> Attitude Controller/4(Airspeed)
  In Bus Element3/1 -> Lateral Guidance Logic/1(Course SP)
  In Bus Element1/1 -> Airspeed-Altitude Controller/1(Airspeed SP)
  In Bus Element20/1 -> Airspeed-Altitude Controller/6(vxyz)
  In Bus Element21/1 -> Airspeed-Altitude Controller/3(Climb Rate SP)
  In Bus Element23/1 -> "Pitch, Airspeed SP from Controller"/3(Airspeed)
  In Bus Element27/1 -> Demux1/1
  Demux1/1 -> Mux4/2
  Demux1/2 -> Mux2/2
  Demux1/3 -> Mux3/2
  In Bus Element17/1 -> Subsystem2/2(pqr)
  In Bus Element26/1 -> Subsystem2/1(Euler)
  Subsystem2/1(Euler Rate) -> Attitude Controller/3(Ang Rate)
  Actuator dT Switch/1 -> Out Bus Element2/1
  Demux/2 -> Out Bus Element/1
  Pitch SP Switch/1 -> [PitchSP], Mux/2
  Airspeed-Altitude Controller/1(Pitch SP) -> Pitch SP Switch/1
  [PitchSP] -> Mux2/1  "ref"
  In Bus Element28/1 -> Mux4/1
  [RollSP] -> Mux3/1  "ref"
  Mux4/1 -> YPR Scope/1  "Yaw Tracking"
  Mux2/1 -> YPR Scope/2  "Pitch Tracking"
  Mux3/1 -> YPR Scope/3  "Roll Tracking"
  Mux5/1 -> Airspeed Altitude Scope/1  "Airspeed Tracking"
  Mux6/1 -> Airspeed Altitude Scope/2  "Altitude Tracking"
  In Bus Element24/1 -> Mux5/1
  In Bus Element29/1 -> Mux5/2
  In Bus Element32/1 -> Selector1/1
  Selector1/1 -> Gain/1
  Gain/1 -> Mux6/2
  In Bus Element33/1 -> Mux6/1  "REF"

== system ab/Autopilot/Multicopter Controller/Altitude Control ==
  note: Maintain altitude previously set when in transition
  Z ref : Inport
  States : Inport  Port=2
  InTransition : Inport  Port=3
  Bus Selector : BusSelector  OutputSignals=Xe,Ve
  Constant : Constant  Value=0
  Gain1 : Gain  Gain=controlParams.D_Z
  NOT : Logic  Operator=NOT  IconShape=distinctive  AllPortsSameDT=off  OutDataTypeStr=boolean
  PID Controller : slpidlib/PID Controller  Controller=P  Form=Parallel  TimeDomain=Discrete-time  UseExternalTs=off  SampleTime=-1  IntegratorMethod=Forward Euler  FilterMethod=Forward Euler  ControllerParametersSource=internal  P=controlParams.P_Z  I=controlParams.I_Z  UseKiTs=off  D=controlParams.D_Z  N=controlParams.N_Z  UseFilter=on  TunerSelectOption=Transfer Function Based (PID Tuner App)  InitialConditionSource=internal  InitialConditionForIntegrator=0  InitialConditionForFilter=0  DifferentiatorICPrevScaledInput=0  ExternalReset=none  TrackingMode=off  Kt=1  LimitOutput=off  SatLimitsSource=internal  UpperSaturationLimit=inf  LowerSaturationLimit=-inf  LinearizeAsGain=on  AntiWindupMode=none  Kb=1  LimitIntegrator=off  UpperIntegratorSaturationLimit=inf  LowerIntegratorSaturationLimit=-inf  POutMin=[]  POutMax=[]  IOutMin=[]  IOutMax=[]  DOutMin=[]  DOutMax=[]  NOutMin=[]  NOutMax=[]  SumOutMin=[]  SumOutMax=[]  SaturationOutMin=[]  SaturationOutMax=[]  PParamMin=[]  PParamMax=[]  IParamMin=[]  IParamMax=[]  DParamMin=[]  DParamMax=[]  NParamMin=[]  NParamMax=[]  KbParamMin=[]  KbParamMax=[]  KtParamMin=[]  KtParamMax=[]  KbOutMin=[]  KbOutMax=[]  KtOutMin=[]  KtOutMax=[]  IntegratorOutMin=[]  IntegratorOutMax=[]  FilterOutMin=[]  FilterOutMax=[]  SumI1OutMin=[]  SumI1OutMax=[]  SumI2OutMin=[]  SumI2OutMax=[]  SumI3OutMin=[]  SumI3OutMax=[]  SumI4OutMin=[]  SumI4OutMax=[]  SumDOutMin=[]  SumDOutMax=[]  DifferentiatorOutMin=[]  DifferentiatorOutMax=[]  FilterDiffOutCoefMin=[]  FilterDiffOutCoefMax=[]  ReciprocalOutMin=[]  ReciprocalOutMax=[]  SumDenOutMin=[]  SumDenOutMax=[]  SumNumOutMin=[]  SumNumOutMax=[]  DivideOutMin=[]  DivideOutMax=[]  UdiffTsProdOutMin=[]  UdiffTsProdOutMax=[]  NTsProdOutMin=[]  NTsProdOutMax=[]  UintegralTsProdOutMin=[]  UintegralTsProdOutMax=[]  UngainTsProdOutMin=[]  UngainTsProdOutMax=[]  ClampingZeroOutDataTypeStr=Inherit: Inherit via back propagation  ClampingZeroOutMin=[]  ClampingZeroOutMax=[]  FilterDenConstantOutDataTypeStr=Inherit: Inherit via back propagation  FilterDenConstantOutMin=[]  FilterDenConstantOutMax=[]  PCopyOutDataTypeStr=Inherit: Inherit via back propagation  PCopyOutMin=[]  PCopyOutMax=[]  NCopyOutDataTypeStr=Inherit: Inherit via back propagation  NCopyOutMin=[]  NCopyOutMax=[]  IntegratorContinuousStateAttributes=''  IntegratorStateMustResolveToSignalObject=off  IntegratorRTWStateStorageClass=Auto  FilterContinuousStateAttributes=''  FilterStateMustResolveToSignalObject=off  FilterRTWStateStorageClass=Auto  ParallelPVariant=InternalParameters  IdealPVariant=Disabled  IVariant=Disabled  DVariant=Disabled  IntegratorVariant=Disabled  SatVariant=Disabled  AWVariant=Disabled  PCopyVariant=Disabled  TRVariant=Disabled  FdbkBlocksVariant=Forward  IdealPFdbkVariant=Disabled  SatFdbkVariant=Disabled  DerivativeFilterVariant=Disabled  NVariant=Disabled  NCopyVariant=Disabled_SignalSpec  FilterICVariant=Disabled  IntegratorICVariant=Disabled  ExternalResetVariant=Disabled  TRSumVariant=Passthrough  SumFdbkVariant=Disabled  SumVariant=Passthrough_P  TsampFilterVariant=InternalTs  TsampNgainVariant=Passthrough  TsampIntegralVariant=Disabled_SignalSpec  ExternalSaturationOutDataTypeStr=Inherit: Same as second input
  PID Controller1 : slpidlib/PID Controller  Controller=PID  Form=Parallel  TimeDomain=Discrete-time  UseExternalTs=off  SampleTime=-1  IntegratorMethod=Forward Euler  FilterMethod=Forward Euler  ControllerParametersSource=internal  P=controlParams.P_VZ  I=controlParams.I_Z  UseKiTs=off  D=controlParams.D_VZ  N=controlParams.N_VZ  UseFilter=on  TunerSelectOption=Transfer Function Based (PID Tuner App)  InitialConditionSource=internal  InitialConditionForIntegrator=0  InitialConditionForFilter=0  DifferentiatorICPrevScaledInput=0  ExternalReset=none  TrackingMode=off  Kt=1  LimitOutput=off  SatLimitsSource=internal  UpperSaturationLimit=inf  LowerSaturationLimit=-inf  LinearizeAsGain=on  AntiWindupMode=none  Kb=1  LimitIntegrator=off  UpperIntegratorSaturationLimit=inf  LowerIntegratorSaturationLimit=-inf  POutMin=[]  POutMax=[]  IOutMin=[]  IOutMax=[]  DOutMin=[]  DOutMax=[]  NOutMin=[]  NOutMax=[]  SumOutMin=[]  SumOutMax=[]  SaturationOutMin=[]  SaturationOutMax=[]  PParamMin=[]  PParamMax=[]  IParamMin=[]  IParamMax=[]  DParamMin=[]  DParamMax=[]  NParamMin=[]  NParamMax=[]  KbParamMin=[]  KbParamMax=[]  KtParamMin=[]  KtParamMax=[]  KbOutMin=[]  KbOutMax=[]  KtOutMin=[]  KtOutMax=[]  IntegratorOutMin=[]  IntegratorOutMax=[]  FilterOutMin=[]  FilterOutMax=[]  SumI1OutMin=[]  SumI1OutMax=[]  SumI2OutMin=[]  SumI2OutMax=[]  SumI3OutMin=[]  SumI3OutMax=[]  SumI4OutMin=[]  SumI4OutMax=[]  SumDOutMin=[]  SumDOutMax=[]  DifferentiatorOutMin=[]  DifferentiatorOutMax=[]  FilterDiffOutCoefMin=[]  FilterDiffOutCoefMax=[]  ReciprocalOutMin=[]  ReciprocalOutMax=[]  SumDenOutMin=[]  SumDenOutMax=[]  SumNumOutMin=[]  SumNumOutMax=[]  DivideOutMin=[]  DivideOutMax=[]  UdiffTsProdOutMin=[]  UdiffTsProdOutMax=[]  NTsProdOutMin=[]  NTsProdOutMax=[]  UintegralTsProdOutMin=[]  UintegralTsProdOutMax=[]  UngainTsProdOutMin=[]  UngainTsProdOutMax=[]  ClampingZeroOutDataTypeStr=Inherit: Inherit via back propagation  ClampingZeroOutMin=[]  ClampingZeroOutMax=[]  FilterDenConstantOutDataTypeStr=Inherit: Inherit via back propagation  FilterDenConstantOutMin=[]  FilterDenConstantOutMax=[]  PCopyOutDataTypeStr=Inherit: Inherit via back propagation  PCopyOutMin=[]  PCopyOutMax=[]  NCopyOutDataTypeStr=Inherit: Inherit via back propagation  NCopyOutMin=[]  NCopyOutMax=[]  IntegratorContinuousStateAttributes=''  IntegratorStateMustResolveToSignalObject=off  IntegratorRTWStateStorageClass=Auto  FilterContinuousStateAttributes=''  FilterStateMustResolveToSignalObject=off  FilterRTWStateStorageClass=Auto  ParallelPVariant=InternalParameters  IdealPVariant=Disabled  IVariant=InternalParameters  DVariant=InternalParameters  IntegratorVariant=Discrete  SatVariant=Disabled  AWVariant=Passthrough  PCopyVariant=Disabled  TRVariant=Disabled  FdbkBlocksVariant=Forward  IdealPFdbkVariant=Disabled  SatFdbkVariant=Disabled  DerivativeFilterVariant=ForwardEulerFilter  NVariant=InternalParameters  NCopyVariant=Disabled  FilterICVariant=InternalICsFilter  IntegratorICVariant=InternalICs  ExternalResetVariant=Disabled  TRSumVariant=Passthrough  SumFdbkVariant=Disabled  SumVariant=Sum_PID  TsampFilterVariant=InternalTs  TsampNgainVariant=Passthrough  TsampIntegralVariant=Disabled_SignalSpec  ExternalSaturationOutDataTypeStr=Inherit: Same as second input
  Rate Limiter : RateLimiter  FallingSlewLimit=-1000  SampleTimeMode=inherited
  Selector : Selector  InputPortWidth=3  IndexOptions=Index vector (dialog)  Indices=[3]  OutputSizes=1
  Selector1 : Selector  InputPortWidth=3  IndexOptions=Index vector (dialog)  Indices=[3]  OutputSizes=1
  Sum : Sum  Inputs=|+-
  Sum1 : Sum  Inputs=|+-
  Sum2 : Sum  Inputs=|++
  Sum3 : Sum  Inputs=|--
  Switch : Switch  Criteria=u2 > Threshold  SaturateOnIntegerOverflow=off  InputSameDT=off
  Triggered Subsystem : Subsystem  TreatAsAtomicUnit=on
  commanded thrust : Outport
  wires:
  Sum/1 -> PID Controller/1
  Z ref/1 -> Switch/1  "Manual"
  States/1 -> Bus Selector/1
  InTransition/1 -> NOT/1, Triggered Subsystem/Trigger
  Switch/1 -> Rate Limiter/1  "Output"
  NOT/1 -> Switch/2
  Triggered Subsystem/1(Reference) -> Switch/3  "Stable"
  Selector/1 -> Sum/2, Triggered Subsystem/1(AltHold)
  Bus Selector/1 -> Selector/1  "<Xe>"
  Bus Selector/2 -> Selector1/1  "<Ve>"
  PID Controller/1 -> Sum2/1
  Selector1/1 -> Sum1/2, Gain1/1
  Gain1/1 -> Sum3/2
  Sum2/1 -> Sum1/1
  Sum1/1 -> PID Controller1/1
  Rate Limiter/1 -> Sum/1
  Sum3/1 -> Sum2/2
  PID Controller1/1 -> commanded thrust/1
  Constant/1 -> Sum3/1

== system ab/Autopilot/Multicopter Controller/Attitude Control ==
  Ref Attitude : Inport
  States : Inport  Port=2
  inTransition : Inport  Port=3
  Attitude Control : Subsystem  VariantControl=AttitudeControl==0
  Derivative Gain : Subsystem  VariantControl=AttitudeControl==1
  Roll torque cmd : Outport
  Pitch torque Cmd : Outport  Port=2
  Yaw torque Cmd : Outport  Port=3

== system ab/Autopilot/Multicopter Controller/Attitude Stabilization ==
  note: Level Tiltrotor when in transition.
  Enable : EnablePort
  Constant : Constant  Value=0
  Constant1 : Constant  Value=0
  Tilt Cmd : Outport
  Roll Cmd : Outport  Port=2
  wires:
  Constant/1 -> Tilt Cmd/1
  Constant1/1 -> Roll Cmd/1

== system ab/Autopilot/Multicopter Controller/Horizontal Position Control ==
  note: Forward Motion is controlled using Tilt.
      | Lateral Motion occurs using roll.
  XRef : Inport
  YRef : Inport  Port=2
  States : Inport  Port=3
  Enable : EnablePort
  Saturation : Saturate  UpperLimit=0.4  LowerLimit=-0.4
  XY Controller : Subsystem
  Roll Cmd : Outport
  Tilt Cmd : Outport  Port=2
  wires:
  XRef/1 -> XY Controller/1(X_ref)
  YRef/1 -> XY Controller/2(Y_ref)
  States/1 -> XY Controller/3(States)
  XY Controller/1(Forward cmd) -> Tilt Cmd/1
  XY Controller/2(Sideward Cmd) -> Saturation/1
  Saturation/1 -> Roll Cmd/1

== system ab/Autopilot/Multicopter Controller/Organize Inputs ==
  forward command : Inport
  commanded phi torque : Inport  Port=2
  commanded theta torque : Inport  Port=3
  commanded psi torque : Inport  Port=4
  commanded thrust : Inport  Port=5
  Out Bus Element : Outport  PortName=MixerCommands  Element=w_phi
  Out Bus Element1 : Outport  PortName=MixerCommands  Element=w_theta
  Out Bus Element2 : Outport  PortName=MixerCommands  Element=l_psi
  Out Bus Element3 : Outport  PortName=MixerCommands  Element=w_z
  Out Bus Element4 : Outport  PortName=MixerCommands  Element=l_x
  tag scope: w_phi=global, w_psi=global, w_theta=global, w_tilt=global, w_z=global
  wires:
  commanded theta torque/1 -> Out Bus Element1/1, [w_theta]  "theta"
  commanded psi torque/1 -> Out Bus Element2/1, [w_psi]  "psi"
  commanded thrust/1 -> Out Bus Element3/1, [w_z]  "thrust"
  forward command/1 -> Out Bus Element4/1, [w_tilt]  "tilt"
  commanded phi torque/1 -> Out Bus Element/1, [w_phi]  "phi"
